simulink library "VSIGenLib"  (R2019b)
settings: Solver=VariableStepAuto  StartTime=0.0  StopTime=10.0  RelTol=1e-3
PostLoadFcn:
  | , if any(exist('dsrtsu_mdlpostloadfcn', 'file') ~= 0), dsrtsu_mdlpostloadfcn('Execute', bdroot); end,
undefined symbols (not defined in the file or in its folder): LIDAR, Ts_hil
libraries: simulink x76, $bdroot x46, etargetslib x30, ASCGenLib x26, dsmpblib x6
(part 3 of 3)

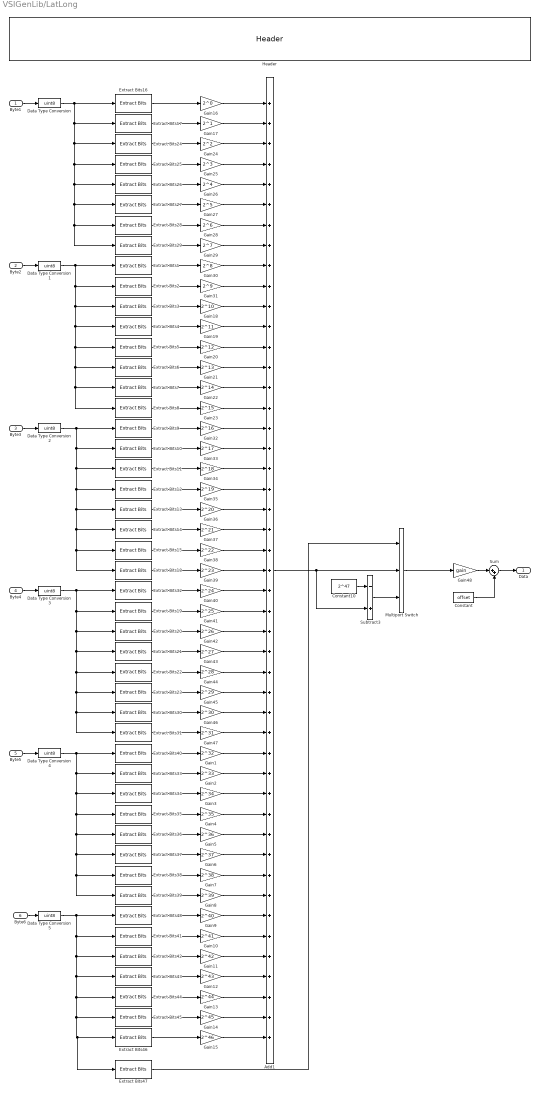
== system VSIGenLib/LatLong ==
  Byte1 : Inport
  Byte2 : Inport  Port=2
  Byte3 : Inport  Port=3
  Byte4 : Inport  Port=4
  Byte5 : Inport  Port=5
  Byte6 : Inport  Port=6
  Add1 : Sum  Inputs=+++++++++++++++++++++++++++++++++++++++++++++++
  Constant : Constant  Value=offset  OutDataTypeStr=double
  Constant10 : Constant  Value=2^47
  Data Type Conversion{,1..5} (6 alike) : DataTypeConversion  OutDataTypeStr=uint8
  Extract Bits{1,9,16,32,40,48} (6 alike) : simulink/Logic and Bit Operations/Extract Bits  bitsToExtract=Range of bits  numBits=8  bitIdxRange=0  outScalingMode=Treat bit field as an integer
      settings: SourceProductName=Simulink
  Extract Bits{2,10,17,19,33,41} (6 alike) : simulink/Logic and Bit Operations/Extract Bits  bitsToExtract=Range of bits  numBits=8  bitIdxRange=1  outScalingMode=Treat bit field as an integer
      settings: SourceProductName=Simulink
  Extract Bits{3,11,20,24,34,42} (6 alike) : simulink/Logic and Bit Operations/Extract Bits  bitsToExtract=Range of bits  numBits=8  bitIdxRange=2  outScalingMode=Treat bit field as an integer
      settings: SourceProductName=Simulink
  Extract Bits{4,12,21,25,35,43} (6 alike) : simulink/Logic and Bit Operations/Extract Bits  bitsToExtract=Range of bits  numBits=8  bitIdxRange=3  outScalingMode=Treat bit field as an integer
      settings: SourceProductName=Simulink
  Extract Bits{5,13,22,26,36,44} (6 alike) : simulink/Logic and Bit Operations/Extract Bits  bitsToExtract=Range of bits  numBits=8  bitIdxRange=4  outScalingMode=Treat bit field as an integer
      settings: SourceProductName=Simulink
  Extract Bits{6,14,23,27,37,45} (6 alike) : simulink/Logic and Bit Operations/Extract Bits  bitsToExtract=Range of bits  numBits=8  bitIdxRange=5  outScalingMode=Treat bit field as an integer
      settings: SourceProductName=Simulink
  Extract Bits{7,15,28,30,38,46} (6 alike) : simulink/Logic and Bit Operations/Extract Bits  bitsToExtract=Range of bits  numBits=8  bitIdxRange=6  outScalingMode=Treat bit field as an integer
      settings: SourceProductName=Simulink
  Extract Bits{8,18,29,31,39,47} (6 alike) : simulink/Logic and Bit Operations/Extract Bits  bitsToExtract=Range of bits  numBits=8  bitIdxRange=7  outScalingMode=Treat bit field as an integer
      settings: SourceProductName=Simulink
  Gain1 : Gain  Gain=2^32  ParamDataTypeStr=double  OutDataTypeStr=double
  Gain10 : Gain  Gain=2^41  ParamDataTypeStr=double  OutDataTypeStr=double
  Gain11 : Gain  Gain=2^42  ParamDataTypeStr=double  OutDataTypeStr=double
  Gain12 : Gain  Gain=2^43  ParamDataTypeStr=double  OutDataTypeStr=double
  Gain13 : Gain  Gain=2^44  ParamDataTypeStr=double  OutDataTypeStr=double
  Gain14 : Gain  Gain=2^45  ParamDataTypeStr=double  OutDataTypeStr=double
  Gain15 : Gain  Gain=2^46  ParamDataTypeStr=double  OutDataTypeStr=double
  Gain16 : Gain  Gain=2^0  ParamDataTypeStr=double  OutDataTypeStr=double
  Gain17 : Gain  Gain=2^1  ParamDataTypeStr=double  OutDataTypeStr=double
  Gain18 : Gain  Gain=2^10  ParamDataTypeStr=double  OutDataTypeStr=double
  Gain19 : Gain  Gain=2^11  ParamDataTypeStr=double  OutDataTypeStr=double
  Gain2 : Gain  Gain=2^33  ParamDataTypeStr=double  OutDataTypeStr=double
  Gain20 : Gain  Gain=2^12  ParamDataTypeStr=double  OutDataTypeStr=double
  Gain21 : Gain  Gain=2^13  ParamDataTypeStr=double  OutDataTypeStr=double
  Gain22 : Gain  Gain=2^14  ParamDataTypeStr=double  OutDataTypeStr=double
  Gain23 : Gain  Gain=2^15  ParamDataTypeStr=double  OutDataTypeStr=double
  Gain24 : Gain  Gain=2^2  ParamDataTypeStr=double  OutDataTypeStr=double
  Gain25 : Gain  Gain=2^3  ParamDataTypeStr=double  OutDataTypeStr=double
  Gain26 : Gain  Gain=2^4  ParamDataTypeStr=double  OutDataTypeStr=double
  Gain27 : Gain  Gain=2^5  ParamDataTypeStr=double  OutDataTypeStr=double
  Gain28 : Gain  Gain=2^6  ParamDataTypeStr=double  OutDataTypeStr=double
  Gain29 : Gain  Gain=2^7  ParamDataTypeStr=double  OutDataTypeStr=double
  Gain3 : Gain  Gain=2^34  ParamDataTypeStr=double  OutDataTypeStr=double
  Gain30 : Gain  Gain=2^8  ParamDataTypeStr=double  OutDataTypeStr=double
  Gain31 : Gain  Gain=2^9  ParamDataTypeStr=double  OutDataTypeStr=double
  Gain32 : Gain  Gain=2^16  ParamDataTypeStr=double  OutDataTypeStr=double
  Gain33 : Gain  Gain=2^17  ParamDataTypeStr=double  OutDataTypeStr=double
  Gain34 : Gain  Gain=2^18  ParamDataTypeStr=double  OutDataTypeStr=double
  Gain35 : Gain  Gain=2^19  ParamDataTypeStr=double  OutDataTypeStr=double
  Gain36 : Gain  Gain=2^20  ParamDataTypeStr=double  OutDataTypeStr=double
  Gain37 : Gain  Gain=2^21  ParamDataTypeStr=double  OutDataTypeStr=double
  Gain38 : Gain  Gain=2^22  ParamDataTypeStr=double  OutDataTypeStr=double
  Gain39 : Gain  Gain=2^23  ParamDataTypeStr=double  OutDataTypeStr=double
  Gain4 : Gain  Gain=2^35  ParamDataTypeStr=double  OutDataTypeStr=double
  Gain40 : Gain  Gain=2^24  ParamDataTypeStr=double  OutDataTypeStr=double
  Gain41 : Gain  Gain=2^25  ParamDataTypeStr=double  OutDataTypeStr=double
  Gain42 : Gain  Gain=2^26  ParamDataTypeStr=double  OutDataTypeStr=double
  Gain43 : Gain  Gain=2^27  ParamDataTypeStr=double  OutDataTypeStr=double
  Gain44 : Gain  Gain=2^28  ParamDataTypeStr=double  OutDataTypeStr=double
  Gain45 : Gain  Gain=2^29  ParamDataTypeStr=double  OutDataTypeStr=double
  Gain46 : Gain  Gain=2^30  ParamDataTypeStr=double  OutDataTypeStr=double
  Gain47 : Gain  Gain=2^31  ParamDataTypeStr=double  OutDataTypeStr=double
  Gain48 : Gain  Gain=gain  ParamDataTypeStr=double  OutDataTypeStr=double
  Gain5 : Gain  Gain=2^36  ParamDataTypeStr=double  OutDataTypeStr=double
  Gain6 : Gain  Gain=2^37  ParamDataTypeStr=double  OutDataTypeStr=double
  Gain7 : Gain  Gain=2^38  ParamDataTypeStr=double  OutDataTypeStr=double
  Gain8 : Gain  Gain=2^39  ParamDataTypeStr=double  OutDataTypeStr=double
  Gain9 : Gain  Gain=2^40  ParamDataTypeStr=double  OutDataTypeStr=double
  Header : $bdroot/Header  not=''
  Multiport Switch : MultiPortSwitch  DataPortOrder=Zero-based contiguous  Inputs=2  zeroidx=on
  Subtract3 : Sum  Inputs=-+
  Sum : Sum  Inputs=|++
  Data : Outport  VectorParamsAs1DForOutWhenUnconnected=off
  wires:
  Extract Bits16/1 -> Gain16/1
  Extract Bits26/1 -> Gain26/1
  Extract Bits27/1 -> Gain27/1
  Extract Bits28/1 -> Gain28/1
  Extract Bits29/1 -> Gain29/1
  Extract Bits1/1 -> Gain30/1
  Extract Bits2/1 -> Gain31/1
  Extract Bits3/1 -> Gain18/1
  Extract Bits4/1 -> Gain19/1
  Extract Bits5/1 -> Gain20/1
  Extract Bits6/1 -> Gain21/1
  Extract Bits7/1 -> Gain22/1
  Extract Bits8/1 -> Gain23/1
  Gain16/1 -> Add1/1
  Gain17/1 -> Add1/2
  Gain24/1 -> Add1/3
  Gain25/1 -> Add1/4
  Gain26/1 -> Add1/5
  Gain27/1 -> Add1/6
  Gain28/1 -> Add1/7
  Gain29/1 -> Add1/8
  Gain30/1 -> Add1/9
  Gain31/1 -> Add1/10
  Gain18/1 -> Add1/11
  Gain19/1 -> Add1/12
  Gain20/1 -> Add1/13
  Gain21/1 -> Add1/14
  Gain22/1 -> Add1/15
  Gain23/1 -> Add1/16
  Extract Bits19/1 -> Gain41/1
  Extract Bits10/1 -> Gain33/1
  Extract Bits20/1 -> Gain42/1
  Extract Bits9/1 -> Gain32/1
  Extract Bits21/1 -> Gain43/1
  Extract Bits11/1 -> Gain34/1
  Extract Bits22/1 -> Gain44/1
  Extract Bits23/1 -> Gain45/1
  Extract Bits30/1 -> Gain46/1
  Extract Bits12/1 -> Gain35/1
  Extract Bits13/1 -> Gain36/1
  Extract Bits14/1 -> Gain37/1
  Extract Bits15/1 -> Gain38/1
  Extract Bits18/1 -> Gain39/1
  Extract Bits32/1 -> Gain40/1
  Extract Bits31/1 -> Gain47/1
  Gain32/1 -> Add1/17
  Gain33/1 -> Add1/18
  Gain34/1 -> Add1/19
  Gain35/1 -> Add1/20
  Gain36/1 -> Add1/21
  Gain37/1 -> Add1/22
  Gain38/1 -> Add1/23
  Gain39/1 -> Add1/24
  Gain40/1 -> Add1/25
  Gain41/1 -> Add1/26
  Gain42/1 -> Add1/27
  Gain43/1 -> Add1/28
  Gain44/1 -> Add1/29
  Gain45/1 -> Add1/30
  Gain46/1 -> Add1/31
  Gain47/1 -> Add1/32
  Byte1/1 -> Data Type Conversion/1
  Byte2/1 -> Data Type Conversion1/1
  Byte3/1 -> Data Type Conversion2/1
  Data Type Conversion3/1 -> Extract Bits19/1, Extract Bits22/1, Extract Bits23/1, Extract Bits30/1, Extract Bits31/1, Extract Bits21/1, Extract Bits20/1, Extract Bits32/1
  Extract Bits33/1 -> Gain2/1
  Extract Bits34/1 -> Gain3/1
  Extract Bits35/1 -> Gain4/1
  Extract Bits36/1 -> Gain5/1
  Extract Bits37/1 -> Gain6/1
  Extract Bits38/1 -> Gain7/1
  Extract Bits40/1 -> Gain1/1
  Extract Bits39/1 -> Gain8/1
  Gain1/1 -> Add1/33
  Gain2/1 -> Add1/34
  Gain3/1 -> Add1/35
  Gain4/1 -> Add1/36
  Gain5/1 -> Add1/37
  Gain6/1 -> Add1/38
  Gain7/1 -> Add1/39
  Gain8/1 -> Add1/40
  Data Type Conversion4/1 -> Extract Bits34/1, Extract Bits35/1, Extract Bits39/1, Extract Bits38/1, Extract Bits37/1, Extract Bits36/1, Extract Bits33/1, Extract Bits40/1
  Extract Bits41/1 -> Gain10/1
  Extract Bits42/1 -> Gain11/1
  Extract Bits43/1 -> Gain12/1
  Extract Bits44/1 -> Gain13/1
  Extract Bits45/1 -> Gain14/1
  Extract Bits46/1 -> Gain15/1
  Extract Bits48/1 -> Gain9/1
  Data Type Conversion5/1 -> Extract Bits48/1, Extract Bits41/1, Extract Bits44/1, Extract Bits45/1, Extract Bits47/1, Extract Bits46/1, Extract Bits43/1, Extract Bits42/1
  Gain15/1 -> Add1/47
  Gain14/1 -> Add1/46
  Gain13/1 -> Add1/45
  Gain12/1 -> Add1/44
  Gain10/1 -> Add1/42
  Gain11/1 -> Add1/43
  Gain9/1 -> Add1/41
  Constant10/1 -> Subtract3/1
  Add1/1 -> Subtract3/2, Multiport Switch/2
  Extract Bits17/1 -> Gain17/1
  Extract Bits25/1 -> Gain25/1
  Extract Bits24/1 -> Gain24/1
  Gain48/1 -> Sum/1
  Constant/1 -> Sum/2
  Multiport Switch/1 -> Gain48/1
  Sum/1 -> Data/1
  Extract Bits47/1 -> Multiport Switch/1
  Subtract3/1 -> Multiport Switch/3
  Data Type Conversion/1 -> Extract Bits17/1, Extract Bits24/1, Extract Bits25/1, Extract Bits27/1, Extract Bits28/1, Extract Bits29/1, Extract Bits26/1, Extract Bits16/1
  Data Type Conversion1/1 -> Extract Bits2/1, Extract Bits3/1, Extract Bits4/1, Extract Bits5/1, Extract Bits6/1, Extract Bits7/1, Extract Bits8/1, Extract Bits1/1
  Data Type Conversion2/1 -> Extract Bits10/1, Extract Bits11/1, Extract Bits12/1, Extract Bits13/1, Extract Bits14/1, Extract Bits15/1, Extract Bits18/1, Extract Bits9/1
  Byte4/1 -> Data Type Conversion3/1
  Byte5/1 -> Data Type Conversion4/1
  Byte6/1 -> Data Type Conversion5/1

== system VSIGenLib/ManualOverride ==
  Data : Inport
  Header : $bdroot/Header  not=''
  Multiport Switch : MultiPortSwitch  Inputs=2
  OvrEnbl : Constant  OutDataTypeStr=boolean
  OvrVal : Constant  Value=0
  "Data " : Outport  VectorParamsAs1DForOutWhenUnconnected=off
  wires:
  Multiport Switch/1 -> "Data "/1
  Data/1 -> Multiport Switch/2
  OvrEnbl/1 -> Multiport Switch/1
  OvrVal/1 -> Multiport Switch/3

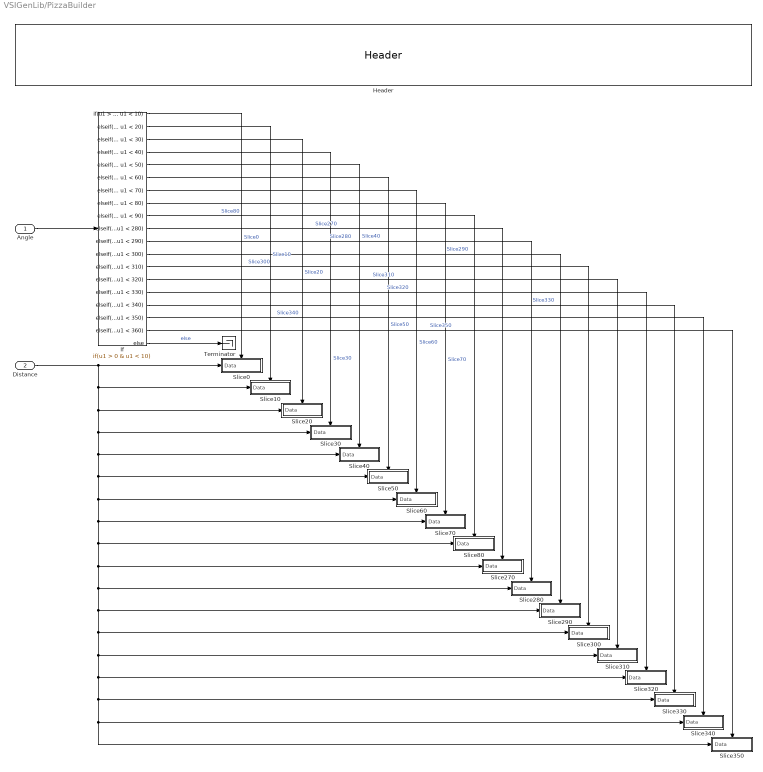
== system VSIGenLib/PizzaBuilder ==
  Angle : Inport
  Distance : Inport  Port=2
  Header : $bdroot/Header  not=''
  If : If  IfExpression=u1 > 0 & u1 < 10  ElseIfExpressions="u1 > 10 & u1 < 20, u1 > 20 & u1 < 30, u1 > 30 & u1 < 40, u1 > 40 & u1 < 50, u1 > 50 & u1 < 60, u1 > 60 & u1 < 70, u1 > 70 & u1 < 80, u1 > 80 & u1 < 90, u1 > 270 & u1 < 280,  u1 > 280 & u1 < 290,  u1 > 290 & u1 < 300,  u1 > 300 & u1 < 310,  u1 > 310 & u1 < 320, u1 > 320 & u1 < 330, u1 > 330 & u1 < 340, u1 > 340 & u1 < 350,  u1 > 350 & u1 < 360"
  Slice0 : Subsystem
  Slice10 : Subsystem
  Slice20 : Subsystem
  Slice270 : Subsystem
  Slice280 : Subsystem
  Slice290 : Subsystem
  Slice30 : Subsystem
  Slice300 : Subsystem
  Slice310 : Subsystem
  Slice320 : Subsystem
  Slice330 : Subsystem
  Slice340 : Subsystem
  Slice350 : Subsystem
  Slice40 : Subsystem
  Slice50 : Subsystem
  Slice60 : Subsystem
  Slice70 : Subsystem
  Slice80 : Subsystem
  Terminator : Terminator
  wires:
  If/19 -> Terminator/1  "else"
  If/18 -> Slice350/Action  "Slice350"
  If/17 -> Slice340/Action  "Slice340"
  If/16 -> Slice330/Action  "Slice330"
  If/15 -> Slice320/Action  "Slice320"
  If/14 -> Slice310/Action  "Slice310"
  If/13 -> Slice300/Action  "Slice300"
  If/12 -> Slice290/Action  "Slice290"
  If/11 -> Slice280/Action  "Slice280"
  If/10 -> Slice270/Action  "Slice270"
  If/9 -> Slice80/Action  "Slice80"
  If/8 -> Slice70/Action  "Slice70"
  If/7 -> Slice60/Action  "Slice60"
  If/6 -> Slice50/Action  "Slice50"
  If/5 -> Slice40/Action  "Slice40"
  If/4 -> Slice30/Action  "Slice30"
  If/3 -> Slice20/Action  "Slice20"
  If/2 -> Slice10/Action  "Slice10"
  If/1 -> Slice0/Action  "Slice0"
  Angle/1 -> If/1
  Distance/1 -> Slice350/1(Data), Slice340/1(Data), Slice330/1(Data), Slice320/1(Data), Slice310/1(Data), Slice300/1(Data), Slice290/1(Data), Slice280/1(Data), Slice270/1(Data), Slice80/1(Data), Slice70/1(Data), Slice60/1(Data), Slice50/1(Data), Slice40/1(Data), Slice30/1(Data), Slice20/1(Data), Slice10/1(Data), Slice0/1(Data)

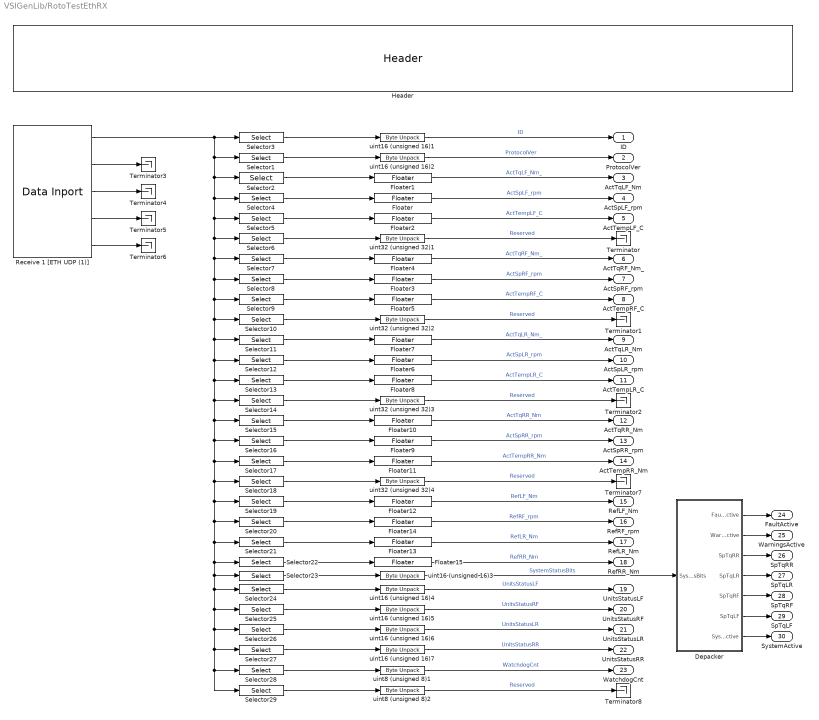
== system VSIGenLib/RotoTestEthRX ==
  Depacker : Subsystem
  Floater{,1..15} (16 alike) : $bdroot/Floater  SystemSampleTime=-1  Latency=0  AutoFrameSizeCalculation=off
  Header : $bdroot/Header  not=''
  Receive 1 [ETH UDP (1)] : dsmpblib/Data Inport  Priority=10000
      settings: SourceProductName=dSPACE Model Interface Blockset
  Selector1 : Selector  IndexMode=Zero-based  InputPortWidth=96  IndexOptions=Index vector (dialog)  Indices=[3 2]  OutputSizes=1
  Selector10 : Selector  IndexMode=Zero-based  InputPortWidth=96  IndexOptions=Index vector (dialog)  Indices=[35 34 33 32]  OutputSizes=1
  Selector11 : Selector  IndexMode=Zero-based  InputPortWidth=96  IndexOptions=Index vector (dialog)  Indices=[39 38 37 36]  OutputSizes=1
  Selector12 : Selector  IndexMode=Zero-based  InputPortWidth=96  IndexOptions=Index vector (dialog)  Indices=[43 42 41 40]  OutputSizes=1
  Selector13 : Selector  IndexMode=Zero-based  InputPortWidth=96  IndexOptions=Index vector (dialog)  Indices=[47 46 45 44]  OutputSizes=1
  Selector14 : Selector  IndexMode=Zero-based  InputPortWidth=96  IndexOptions=Index vector (dialog)  Indices=[51 50 49 48]  OutputSizes=1
  Selector15 : Selector  IndexMode=Zero-based  InputPortWidth=96  IndexOptions=Index vector (dialog)  Indices=[55 54 53 52]  OutputSizes=1
  Selector16 : Selector  IndexMode=Zero-based  InputPortWidth=96  IndexOptions=Index vector (dialog)  Indices=[59 58 57 56]  OutputSizes=1
  Selector17 : Selector  IndexMode=Zero-based  InputPortWidth=96  IndexOptions=Index vector (dialog)  Indices=[63 62 61 60]  OutputSizes=1
  Selector18 : Selector  IndexMode=Zero-based  InputPortWidth=96  IndexOptions=Index vector (dialog)  Indices=[67 66 65 64]  OutputSizes=1
  Selector19 : Selector  IndexMode=Zero-based  InputPortWidth=96  IndexOptions=Index vector (dialog)  Indices=[71 70 69 68]  OutputSizes=1
  Selector2 : Selector  IndexMode=Zero-based  InputPortWidth=96  IndexOptions=Index vector (dialog)  Indices=[7 6 5 4]  OutputSizes=1
  Selector20 : Selector  IndexMode=Zero-based  InputPortWidth=96  IndexOptions=Index vector (dialog)  Indices=[75 74 73 72]  OutputSizes=1
  Selector21 : Selector  IndexMode=Zero-based  InputPortWidth=96  IndexOptions=Index vector (dialog)  Indices=[79 78 77 76]  OutputSizes=1
  Selector22 : Selector  IndexMode=Zero-based  InputPortWidth=96  IndexOptions=Index vector (dialog)  Indices=[83 82 81 80]  OutputSizes=1
  Selector23 : Selector  IndexMode=Zero-based  InputPortWidth=96  IndexOptions=Index vector (dialog)  Indices=[85 84]  OutputSizes=1
  Selector24 : Selector  IndexMode=Zero-based  InputPortWidth=96  IndexOptions=Index vector (dialog)  Indices=[87 86]  OutputSizes=1
  Selector25 : Selector  IndexMode=Zero-based  InputPortWidth=96  IndexOptions=Index vector (dialog)  Indices=[89 88]  OutputSizes=1
  Selector26 : Selector  IndexMode=Zero-based  InputPortWidth=96  IndexOptions=Index vector (dialog)  Indices=[91 90]  OutputSizes=1
  Selector27 : Selector  IndexMode=Zero-based  InputPortWidth=96  IndexOptions=Index vector (dialog)  Indices=[93 92]  OutputSizes=1
  Selector28 : Selector  IndexMode=Zero-based  InputPortWidth=96  IndexOptions=Index vector (dialog)  Indices=[94]  OutputSizes=1
  Selector29 : Selector  IndexMode=Zero-based  InputPortWidth=96  IndexOptions=Index vector (dialog)  Indices=[95]  OutputSizes=1
  Selector3 : Selector  IndexMode=Zero-based  InputPortWidth=96  IndexOptions=Index vector (dialog)  Indices=[1 0]  OutputSizes=1
  Selector4 : Selector  IndexMode=Zero-based  InputPortWidth=96  IndexOptions=Index vector (dialog)  Indices=[11 10 9 8]  OutputSizes=1
  Selector5 : Selector  IndexMode=Zero-based  InputPortWidth=96  IndexOptions=Index vector (dialog)  Indices=[15 14 13 12]  OutputSizes=1
  Selector6 : Selector  IndexMode=Zero-based  InputPortWidth=96  IndexOptions=Index vector (dialog)  Indices=[19 18 17 16]  OutputSizes=1
  Selector7 : Selector  IndexMode=Zero-based  InputPortWidth=96  IndexOptions=Index vector (dialog)  Indices=[23 22 21 20]  OutputSizes=1
  Selector8 : Selector  IndexMode=Zero-based  InputPortWidth=96  IndexOptions=Index vector (dialog)  Indices=[27 26 25 24]  OutputSizes=1
  Selector9 : Selector  IndexMode=Zero-based  InputPortWidth=96  IndexOptions=Index vector (dialog)  Indices=[31 30 29 28]  OutputSizes=1
  Terminator{,1..8} (9 alike) : Terminator
  uint16 (unsigned 16){1..7} (7 alike) : etargetslib/Byte Unpack  dimensions={[1]}  datatypes={'uint16'}  byteAlign=1
      settings: SourceProductName=MATLAB Coder
  uint32 (unsigned 32){1..4} (4 alike) : etargetslib/Byte Unpack  dimensions={[1]}  datatypes={'uint32'}  byteAlign=1
      settings: SourceProductName=MATLAB Coder
  uint8 (unsigned 8)1 : etargetslib/Byte Unpack  dimensions={[1]}  datatypes={'uint8'}  byteAlign=1
      settings: SourceProductName=MATLAB Coder
  uint8 (unsigned 8)2 : etargetslib/Byte Unpack  dimensions={[1]}  datatypes={'uint8'}  byteAlign=1
      settings: SourceProductName=MATLAB Coder
  ID : Outport
  ProtocolVer : Outport  Port=2
  ActTqLF_Nm : Outport  Port=3
  ActSpLF_rpm : Outport  Port=4
  ActTempLF_C : Outport  Port=5
  ActTqRF_Nm_ : Outport  Port=6
  ActSpRF_rpm : Outport  Port=7
  ActTempRF_C : Outport  Port=8
  ActTqLR_Nm : Outport  Port=9
  ActSpLR_rpm : Outport  Port=10
  ActTempLR_C : Outport  Port=11
  ActTqRR_Nm : Outport  Port=12
  ActSpRR_rpm : Outport  Port=13
  ActTempRR_Nm : Outport  Port=14
  RefLF_Nm : Outport  Port=15
  RefRF_rpm : Outport  Port=16
  RefLR_Nm : Outport  Port=17
  RefRR_Nm : Outport  Port=18
  UnitsStatusLF : Outport  Port=19
  UnitsStatusRF : Outport  Port=20
  UnitsStatusLR : Outport  Port=21
  UnitsStatusRR : Outport  Port=22
  WatchdogCnt : Outport  Port=23
  FaultActive : Outport  Port=24
  WarningsActive : Outport  Port=25
  SpTqRR : Outport  Port=26
  SpTqLR : Outport  Port=27
  SpTqRF : Outport  Port=28
  SpTqLF : Outport  Port=29
  SystemActive : Outport  Port=30
  wires:
  Depacker/7(SystemActive) -> SystemActive/1
  Depacker/5(SpTqRF) -> SpTqRF/1
  Depacker/1(FaultActive) -> FaultActive/1
  Depacker/2(WarningsActive) -> WarningsActive/1
  Depacker/3(SpTqRR) -> SpTqRR/1
  Depacker/4(SpTqLR) -> SpTqLR/1
  Depacker/6(SpTqLF) -> SpTqLF/1
  Floater5/1 -> ActTempRF_C/1  "ActTempRF_C"
  uint32 (unsigned 32)2/1 -> Terminator1/1  "Reserved"
  Floater/1 -> ActSpLF_rpm/1  "ActSpLF_rpm"
  uint32 (unsigned 32)1/1 -> Terminator/1  "Reserved"
  uint16 (unsigned 16)1/1 -> ID/1  "ID"
  Floater15/1 -> RefRR_Nm/1  "RefRR_Nm"
  uint8 (unsigned 8)1/1 -> WatchdogCnt/1  "WatchdogCnt"
  Floater14/1 -> RefRF_rpm/1  "RefRF_rpm"
  uint16 (unsigned 16)5/1 -> UnitsStatusRF/1  "UnitsStatusRF"
  uint32 (unsigned 32)3/1 -> Terminator2/1  "Reserved"
  Floater9/1 -> ActSpRR_rpm/1  "ActSpRR_rpm"
  Floater1/1 -> ActTqLF_Nm/1  "ActTqLF_Nm_"
  Floater2/1 -> ActTempLF_C/1  "ActTempLF_C"
  Floater12/1 -> RefLF_Nm/1  "RefLF_Nm"
  Floater7/1 -> ActTqLR_Nm/1  "ActTqLR_Nm_"
  uint16 (unsigned 16)2/1 -> ProtocolVer/1  "ProtocolVer"
  Selector24/1 -> uint16 (unsigned 16)4/1
  Selector7/1 -> Floater4/1
  Selector8/1 -> Floater3/1
  uint16 (unsigned 16)7/1 -> UnitsStatusRR/1  "UnitsStatusRR"
  Selector22/1 -> Floater15/1
  Selector18/1 -> uint32 (unsigned 32)4/1
  Selector12/1 -> Floater6/1
  Selector23/1 -> uint16 (unsigned 16)3/1
  uint16 (unsigned 16)6/1 -> UnitsStatusLR/1  "UnitsStatusLR"
  Selector17/1 -> Floater11/1
  Receive 1 [ETH UDP (1)]/3 -> Terminator4/1
  uint16 (unsigned 16)4/1 -> UnitsStatusLF/1  "UnitsStatusLF"
  Selector27/1 -> uint16 (unsigned 16)7/1
  Floater13/1 -> RefLR_Nm/1  "RefLR_Nm"
  Selector14/1 -> uint32 (unsigned 32)3/1
  Selector2/1 -> Floater1/1
  Selector13/1 -> Floater8/1
  Selector26/1 -> uint16 (unsigned 16)6/1
  Selector6/1 -> uint32 (unsigned 32)1/1
  uint16 (unsigned 16)3/1 -> Depacker/1(SysStsBits)  "SystemStatusBits"
  uint32 (unsigned 32)4/1 -> Terminator7/1  "Reserved"
  Floater3/1 -> ActSpRF_rpm/1  "ActSpRF_rpm"
  Receive 1 [ETH UDP (1)]/2 -> Terminator3/1
  Selector25/1 -> uint16 (unsigned 16)5/1
  Floater4/1 -> ActTqRF_Nm_/1  "ActTqRF_Nm_"
  uint8 (unsigned 8)2/1 -> Terminator8/1  "Reserved"
  Floater11/1 -> ActTempRR_Nm/1  "ActTempRR_Nm"
  Floater6/1 -> ActSpLR_rpm/1  "ActSpLR_rpm"
  Selector20/1 -> Floater14/1
  Selector9/1 -> Floater5/1
  Selector5/1 -> Floater2/1
  Selector15/1 -> Floater10/1
  Selector16/1 -> Floater9/1
  Floater8/1 -> ActTempLR_C/1  "ActTempLR_C"
  Selector3/1 -> uint16 (unsigned 16)1/1
  Receive 1 [ETH UDP (1)]/4 -> Terminator5/1
  Selector28/1 -> uint8 (unsigned 8)1/1
  Selector29/1 -> uint8 (unsigned 8)2/1
  Selector21/1 -> Floater13/1
  Receive 1 [ETH UDP (1)]/1 -> Selector7/1, Selector8/1, Selector9/1, Selector10/1, Selector11/1, Selector12/1, Selector13/1, Selector17/1, Selector18/1, Selector19/1, Selector20/1, Selector21/1, Selector22/1, Selector23/1, Selector25/1, Selector26/1, Selector27/1, Selector29/1, Selector28/1, Selector24/1, Selector16/1, Selector15/1, Selector14/1, Selector6/1, Selector5/1, Selector4/1, Selector2/1, Selector1/1, Selector3/1
  Selector19/1 -> Floater12/1
  Selector10/1 -> uint32 (unsigned 32)2/1
  Selector1/1 -> uint16 (unsigned 16)2/1
  Receive 1 [ETH UDP (1)]/5 -> Terminator6/1
  Selector4/1 -> Floater/1
  Floater10/1 -> ActTqRR_Nm/1  "ActTqRR_Nm"
  Selector11/1 -> Floater7/1

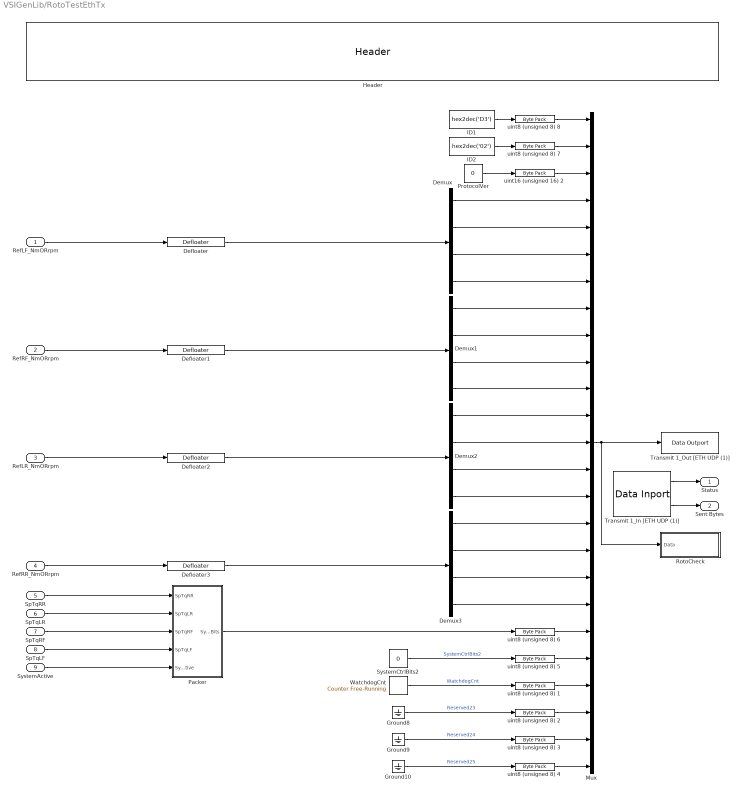
== system VSIGenLib/RotoTestEthTx ==
  RefLF_NmORrpm : Inport
  RefRF_NmORrpm : Inport  Port=2
  RefLR_NmORrpm : Inport  Port=3
  RefRR_NmORrpm : Inport  Port=4
  SpTqRR : Inport  Port=5
  SpTqLR : Inport  Port=6
  SpTqRF : Inport  Port=7
  SpTqLF : Inport  Port=8
  SystemActive : Inport  Port=9
  Defloater{,1..3} (4 alike) : $bdroot/Defloater  SystemSampleTime=-1  Latency=0  AutoFrameSizeCalculation=off
  Demux{,1..3} (4 alike) : Demux
  Ground10 : Ground
  Ground8 : Ground
  Ground9 : Ground
  Header : $bdroot/Header  not=''
  ID1 : Constant  Value=hex2dec('D3')  OutDataTypeStr=uint8
  ID2 : Constant  Value=hex2dec('02')  OutDataTypeStr=uint8
  Mux : Mux  Inputs=25
  Packer : Subsystem
  ProtocolVer : Constant  Value=0  OutDataTypeStr=uint16
  RotoCheck : Subsystem
  SystemCtrlBits2 : Constant  Value=0  OutDataTypeStr=uint8
  Transmit 1_In [ETH UDP (1)] : dsmpblib/Data Inport  Priority=10000
      settings: SourceProductName=dSPACE Model Interface Blockset
  Transmit 1_Out [ETH UDP (1)] : dsmpblib/Data Outport  Priority=-10000
      settings: SourceProductName=dSPACE Model Interface Blockset
  WatchdogCnt : simulink/Sources/Counter Free-Running  NumBits=8  tsamp=-1
  uint16 (unsigned 16) 2 : etargetslib/Byte Pack  datatypes={'uint16'}  byteAlign=1
      settings: SourceProductName=MATLAB Coder
  uint8 (unsigned 8) {1..8} (8 alike) : etargetslib/Byte Pack  datatypes={'uint8'}  byteAlign=1
      settings: SourceProductName=MATLAB Coder
  Status : Outport
  Sent Bytes : Outport  Port=2
  wires:
  Transmit 1_In [ETH UDP (1)]/2 -> Sent Bytes/1
  Transmit 1_In [ETH UDP (1)]/1 -> Status/1
  Packer/1(SystemCtrlBits) -> uint8 (unsigned 8) 6/1
  SystemActive/1 -> Packer/5(SystemActive)
  SpTqLF/1 -> Packer/4(SpTqLF)
  SpTqRF/1 -> Packer/3(SpTqRF)
  SpTqLR/1 -> Packer/2(SpTqLR)
  SpTqRR/1 -> Packer/1(SpTqRR)
  RefLR_NmORrpm/1 -> Defloater2/1
  RefLF_NmORrpm/1 -> Defloater/1
  Demux3/2 -> Mux/17
  Ground8/1 -> uint8 (unsigned 8) 2/1  "Reserved23"
  Demux/2 -> Mux/5
  RefRR_NmORrpm/1 -> Defloater3/1
  uint8 (unsigned 8) 7/1 -> Mux/2
  SystemCtrlBits2/1 -> uint8 (unsigned 8) 5/1  "SystemCtrlBits2"
  Demux3/4 -> Mux/19
  Demux2/4 -> Mux/15
  uint8 (unsigned 8) 8/1 -> Mux/1
  Mux/1 -> Transmit 1_Out [ETH UDP (1)]/1, RotoCheck/1(Data)
  Demux/3 -> Mux/6
  Demux1/2 -> Mux/9
  uint8 (unsigned 8) 6/1 -> Mux/20
  Demux2/3 -> Mux/14
  Demux/4 -> Mux/7
  Demux2/1 -> Mux/12
  Defloater/1 -> Demux/1
  Defloater1/1 -> Demux1/1
  uint16 (unsigned 16) 2/1 -> Mux/3
  uint8 (unsigned 8) 1/1 -> Mux/22
  Demux2/2 -> Mux/13
  uint8 (unsigned 8) 3/1 -> Mux/24
  ProtocolVer/1 -> uint16 (unsigned 16) 2/1
  Demux1/1 -> Mux/8
  Demux3/1 -> Mux/16
  Demux/1 -> Mux/4
  uint8 (unsigned 8) 4/1 -> Mux/25
  ID1/1 -> uint8 (unsigned 8) 8/1
  Ground9/1 -> uint8 (unsigned 8) 3/1  "Reserved24"
  uint8 (unsigned 8) 2/1 -> Mux/23
  Demux1/3 -> Mux/10
  uint8 (unsigned 8) 5/1 -> Mux/21
  Demux3/3 -> Mux/18
  Defloater3/1 -> Demux3/1
  WatchdogCnt/1 -> uint8 (unsigned 8) 1/1  "WatchdogCnt"
  Ground10/1 -> uint8 (unsigned 8) 4/1  "Reserved25"
  Demux1/4 -> Mux/11
  RefRF_NmORrpm/1 -> Defloater1/1
  ID2/1 -> uint8 (unsigned 8) 7/1
  Defloater2/1 -> Demux2/1

== system VSIGenLib/SmartFilter ==
  Slice : Inport
  Tau : Inport  Port=2
  AgeCheck : Stateflow chart  TreatAsAtomicUnit=on
  AgeCheck1 : Stateflow chart  TreatAsAtomicUnit=on
  AgeCheck10 : Stateflow chart  TreatAsAtomicUnit=on
  AgeCheck11 : Stateflow chart  TreatAsAtomicUnit=on
  AgeCheck2 : Stateflow chart  TreatAsAtomicUnit=on
  AgeCheck3 : Stateflow chart  TreatAsAtomicUnit=on
  AgeCheck4 : Stateflow chart  TreatAsAtomicUnit=on
  AgeCheck5 : Stateflow chart  TreatAsAtomicUnit=on
  AgeCheck6 : Stateflow chart  TreatAsAtomicUnit=on
  AgeCheck7 : Stateflow chart  TreatAsAtomicUnit=on
  AgeCheck8 : Stateflow chart  TreatAsAtomicUnit=on
  AgeCheck9 : Stateflow chart  TreatAsAtomicUnit=on
  Demux : Demux  Outputs=12
  FirstOrderFilterTau : $bdroot/FirstOrderFilterTau  SystemSampleTime=-1  Latency=0  AutoFrameSizeCalculation=off
  Header : $bdroot/Header  not=''
  MinMax : MinMax  Inputs=12
  SliceMin : Outport  VectorParamsAs1DForOutWhenUnconnected=off
  wires:
  Demux/1 -> AgeCheck/1(In)
  AgeCheck/1(Out) -> MinMax/1
  Slice/1 -> Demux/1
  MinMax/1 -> FirstOrderFilterTau/1
  Demux/2 -> AgeCheck1/1(In)
  Demux/3 -> AgeCheck2/1(In)
  Demux/4 -> AgeCheck3/1(In)
  Demux/5 -> AgeCheck4/1(In)
  Demux/6 -> AgeCheck5/1(In)
  Demux/7 -> AgeCheck6/1(In)
  Demux/8 -> AgeCheck7/1(In)
  Demux/9 -> AgeCheck8/1(In)
  Demux/10 -> AgeCheck9/1(In)
  Demux/11 -> AgeCheck10/1(In)
  Demux/12 -> AgeCheck11/1(In)
  AgeCheck1/1(Out) -> MinMax/2
  AgeCheck2/1(Out) -> MinMax/3
  AgeCheck3/1(Out) -> MinMax/4
  AgeCheck4/1(Out) -> MinMax/5
  AgeCheck5/1(Out) -> MinMax/6
  AgeCheck6/1(Out) -> MinMax/7
  AgeCheck7/1(Out) -> MinMax/8
  AgeCheck8/1(Out) -> MinMax/9
  AgeCheck9/1(Out) -> MinMax/10
  AgeCheck10/1(Out) -> MinMax/11
  AgeCheck11/1(Out) -> MinMax/12
  Tau/1 -> FirstOrderFilterTau/2
  FirstOrderFilterTau/1 -> SliceMin/1

== system VSIGenLib/Timer ==
  Start : Inport
  Header : $bdroot/Header  not=''
  Memory : Memory  InheritSampleTime=on
  Sum : Sum  Inputs=|++
  Switch : Switch  Criteria=u2 ~= 0
  Ts_hil : Constant  Value=Ts_hil
  Zero : Constant  Value=0
  Timer : Outport  VectorParamsAs1DForOutWhenUnconnected=off
  wires:
  Ts_hil/1 -> Sum/1
  Sum/1 -> Switch/1
  Memory/1 -> Timer/1, Sum/2
  Zero/1 -> Switch/3
  Start/1 -> Switch/2
  Switch/1 -> Memory/1

== system VSIGenLib/PizzaBuilder/Slice0 ==
  Data : Inport
  Action Port : ActionPort  ActionPortLabel=if { }
  CANRxEnblWrite : DataStoreWrite  DataStoreName=Slice0
  Header : ASCGenLib/Header  not=''
  wires:
  Data/1 -> CANRxEnblWrite/1

== system VSIGenLib/PizzaBuilder/Slice10 ==
  Data : Inport
  Action Port : ActionPort  ActionPortLabel=elseif { }
  CANRxEnblWrite : DataStoreWrite  DataStoreName=Slice10
  Header : ASCGenLib/Header  not=''
  wires:
  Data/1 -> CANRxEnblWrite/1

== system VSIGenLib/PizzaBuilder/Slice20 ==
  Data : Inport
  Action Port : ActionPort  ActionPortLabel=elseif { }
  CANRxEnblWrite : DataStoreWrite  DataStoreName=Slice20
  Header : ASCGenLib/Header  not=''
  wires:
  Data/1 -> CANRxEnblWrite/1

== system VSIGenLib/PizzaBuilder/Slice270 ==
  Data : Inport
  Action Port : ActionPort  ActionPortLabel=elseif { }
  CANRxEnblWrite : DataStoreWrite  DataStoreName=Slice270
  Header : ASCGenLib/Header  not=''
  wires:
  Data/1 -> CANRxEnblWrite/1

== system VSIGenLib/PizzaBuilder/Slice280 ==
  Data : Inport
  Action Port : ActionPort  ActionPortLabel=elseif { }
  CANRxEnblWrite : DataStoreWrite  DataStoreName=Slice280
  Header : ASCGenLib/Header  not=''
  wires:
  Data/1 -> CANRxEnblWrite/1

== system VSIGenLib/PizzaBuilder/Slice290 ==
  Data : Inport
  Action Port : ActionPort  ActionPortLabel=elseif { }
  CANRxEnblWrite : DataStoreWrite  DataStoreName=Slice290
  Header : ASCGenLib/Header  not=''
  wires:
  Data/1 -> CANRxEnblWrite/1

== system VSIGenLib/PizzaBuilder/Slice30 ==
  Data : Inport
  Action Port : ActionPort  ActionPortLabel=elseif { }
  CANRxEnblWrite : DataStoreWrite  DataStoreName=Slice30
  Header : ASCGenLib/Header  not=''
  wires:
  Data/1 -> CANRxEnblWrite/1

== system VSIGenLib/PizzaBuilder/Slice300 ==
  Data : Inport
  Action Port : ActionPort  ActionPortLabel=elseif { }
  CANRxEnblWrite : DataStoreWrite  DataStoreName=Slice300
  Header : ASCGenLib/Header  not=''
  wires:
  Data/1 -> CANRxEnblWrite/1

== system VSIGenLib/PizzaBuilder/Slice310 ==
  Data : Inport
  Action Port : ActionPort  ActionPortLabel=elseif { }
  CANRxEnblWrite : DataStoreWrite  DataStoreName=Slice310
  Header : ASCGenLib/Header  not=''
  wires:
  Data/1 -> CANRxEnblWrite/1

== system VSIGenLib/PizzaBuilder/Slice320 ==
  Data : Inport
  Action Port : ActionPort  ActionPortLabel=elseif { }
  CANRxEnblWrite : DataStoreWrite  DataStoreName=Slice320
  Header : ASCGenLib/Header  not=''
  wires:
  Data/1 -> CANRxEnblWrite/1

== system VSIGenLib/PizzaBuilder/Slice330 ==
  Data : Inport
  Action Port : ActionPort  ActionPortLabel=elseif { }
  CANRxEnblWrite : DataStoreWrite  DataStoreName=Slice330
  Header : ASCGenLib/Header  not=''
  wires:
  Data/1 -> CANRxEnblWrite/1

== system VSIGenLib/PizzaBuilder/Slice340 ==
  Data : Inport
  Action Port : ActionPort  ActionPortLabel=elseif { }
  CANRxEnblWrite : DataStoreWrite  DataStoreName=Slice340
  Header : ASCGenLib/Header  not=''
  wires:
  Data/1 -> CANRxEnblWrite/1

== system VSIGenLib/PizzaBuilder/Slice350 ==
  Data : Inport
  Action Port : ActionPort  ActionPortLabel=elseif { }
  CANRxEnblWrite : DataStoreWrite  DataStoreName=Slice350
  Header : ASCGenLib/Header  not=''
  wires:
  Data/1 -> CANRxEnblWrite/1

== system VSIGenLib/PizzaBuilder/Slice40 ==
  Data : Inport
  Action Port : ActionPort  ActionPortLabel=elseif { }
  CANRxEnblWrite : DataStoreWrite  DataStoreName=Slice40
  Header : ASCGenLib/Header  not=''
  wires:
  Data/1 -> CANRxEnblWrite/1

== system VSIGenLib/PizzaBuilder/Slice50 ==
  Data : Inport
  Action Port : ActionPort  ActionPortLabel=elseif { }
  CANRxEnblWrite : DataStoreWrite  DataStoreName=Slice50
  Header : ASCGenLib/Header  not=''
  wires:
  Data/1 -> CANRxEnblWrite/1

== system VSIGenLib/PizzaBuilder/Slice60 ==
  Data : Inport
  Action Port : ActionPort  ActionPortLabel=elseif { }
  CANRxEnblWrite : DataStoreWrite  DataStoreName=Slice60
  Header : ASCGenLib/Header  not=''
  wires:
  Data/1 -> CANRxEnblWrite/1

== system VSIGenLib/PizzaBuilder/Slice70 ==
  Data : Inport
  Action Port : ActionPort  ActionPortLabel=elseif { }
  CANRxEnblWrite : DataStoreWrite  DataStoreName=Slice70
  Header : ASCGenLib/Header  not=''
  wires:
  Data/1 -> CANRxEnblWrite/1

== system VSIGenLib/PizzaBuilder/Slice80 ==
  Data : Inport
  Action Port : ActionPort  ActionPortLabel=elseif { }
  CANRxEnblWrite : DataStoreWrite  DataStoreName=Slice80
  Header : ASCGenLib/Header  not=''
  wires:
  Data/1 -> CANRxEnblWrite/1

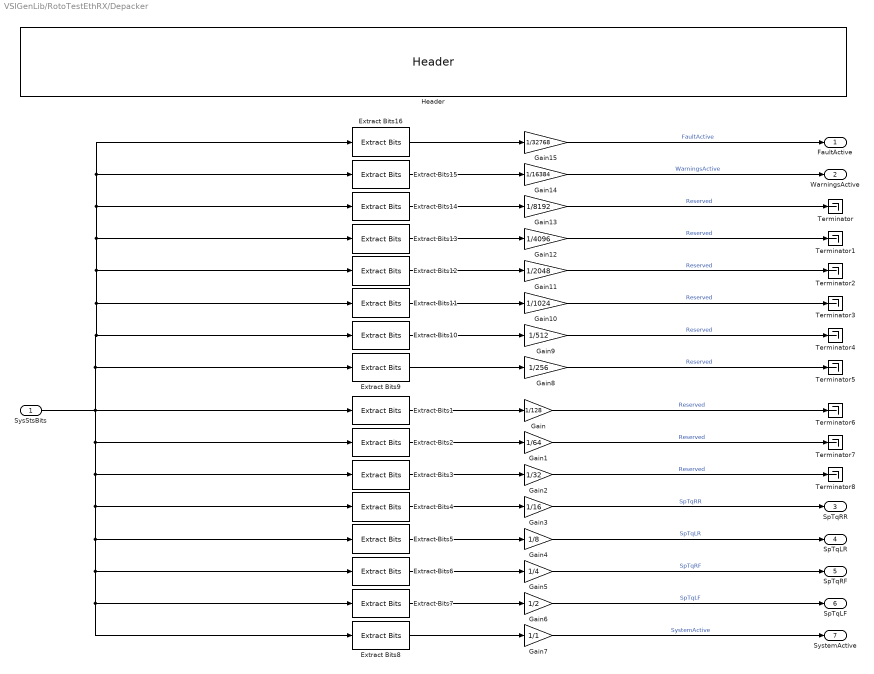
== system VSIGenLib/RotoTestEthRX/Depacker ==
  SysStsBits : Inport
  Extract Bits1 : simulink/Logic and Bit Operations/Extract Bits  bitsToExtract=Range of bits  numBits=8  bitIdxRange=[7]  outScalingMode=Preserve fixed-point scaling
      settings: SourceProductName=Simulink
  Extract Bits10 : simulink/Logic and Bit Operations/Extract Bits  bitsToExtract=Range of bits  numBits=8  bitIdxRange=[9]  outScalingMode=Preserve fixed-point scaling
      settings: SourceProductName=Simulink
  Extract Bits11 : simulink/Logic and Bit Operations/Extract Bits  bitsToExtract=Range of bits  numBits=8  bitIdxRange=[10]  outScalingMode=Preserve fixed-point scaling
      settings: SourceProductName=Simulink
  Extract Bits12 : simulink/Logic and Bit Operations/Extract Bits  bitsToExtract=Range of bits  numBits=8  bitIdxRange=[11]  outScalingMode=Preserve fixed-point scaling
      settings: SourceProductName=Simulink
  Extract Bits13 : simulink/Logic and Bit Operations/Extract Bits  bitsToExtract=Range of bits  numBits=8  bitIdxRange=[12]  outScalingMode=Preserve fixed-point scaling
      settings: SourceProductName=Simulink
  Extract Bits14 : simulink/Logic and Bit Operations/Extract Bits  bitsToExtract=Range of bits  numBits=8  bitIdxRange=[13]  outScalingMode=Preserve fixed-point scaling
      settings: SourceProductName=Simulink
  Extract Bits15 : simulink/Logic and Bit Operations/Extract Bits  bitsToExtract=Range of bits  numBits=8  bitIdxRange=[14]  outScalingMode=Preserve fixed-point scaling
      settings: SourceProductName=Simulink
  Extract Bits16 : simulink/Logic and Bit Operations/Extract Bits  bitsToExtract=Range of bits  numBits=8  bitIdxRange=[15]  outScalingMode=Preserve fixed-point scaling
      settings: SourceProductName=Simulink
  Extract Bits2 : simulink/Logic and Bit Operations/Extract Bits  bitsToExtract=Range of bits  numBits=8  bitIdxRange=[6]  outScalingMode=Preserve fixed-point scaling
      settings: SourceProductName=Simulink
  Extract Bits3 : simulink/Logic and Bit Operations/Extract Bits  bitsToExtract=Range of bits  numBits=8  bitIdxRange=[5]  outScalingMode=Preserve fixed-point scaling
      settings: SourceProductName=Simulink
  Extract Bits4 : simulink/Logic and Bit Operations/Extract Bits  bitsToExtract=Range of bits  numBits=8  bitIdxRange=[4]  outScalingMode=Preserve fixed-point scaling
      settings: SourceProductName=Simulink
  Extract Bits5 : simulink/Logic and Bit Operations/Extract Bits  bitsToExtract=Range of bits  numBits=8  bitIdxRange=[3]  outScalingMode=Preserve fixed-point scaling
      settings: SourceProductName=Simulink
  Extract Bits6 : simulink/Logic and Bit Operations/Extract Bits  bitsToExtract=Range of bits  numBits=8  bitIdxRange=[2]  outScalingMode=Preserve fixed-point scaling
      settings: SourceProductName=Simulink
  Extract Bits7 : simulink/Logic and Bit Operations/Extract Bits  bitsToExtract=Range of bits  numBits=8  bitIdxRange=[1]  outScalingMode=Preserve fixed-point scaling
      settings: SourceProductName=Simulink
  Extract Bits8 : simulink/Logic and Bit Operations/Extract Bits  bitsToExtract=Range of bits  numBits=8  bitIdxRange=[0]  outScalingMode=Preserve fixed-point scaling
      settings: SourceProductName=Simulink
  Extract Bits9 : simulink/Logic and Bit Operations/Extract Bits  bitsToExtract=Range of bits  numBits=8  bitIdxRange=[8]  outScalingMode=Preserve fixed-point scaling
      settings: SourceProductName=Simulink
  Gain : Gain  Gain=1/128
  Gain1 : Gain  Gain=1/64
  Gain10 : Gain  Gain=1/1024
  Gain11 : Gain  Gain=1/2048
  Gain12 : Gain  Gain=1/4096
  Gain13 : Gain  Gain=1/8192
  Gain14 : Gain  Gain=1/16384
  Gain15 : Gain  Gain=1/32768
  Gain2 : Gain  Gain=1/32
  Gain3 : Gain  Gain=1/16
  Gain4 : Gain  Gain=1/8
  Gain5 : Gain  Gain=1/4
  Gain6 : Gain  Gain=1/2
  Gain7 : Gain  Gain=1/1
  Gain8 : Gain  Gain=1/256
  Gain9 : Gain  Gain=1/512
  Header : $bdroot/Header  not=''
  Terminator{,1..8} (9 alike) : Terminator
  FaultActive : Outport
  WarningsActive : Outport  Port=2
  SpTqRR : Outport  Port=3
  SpTqLR : Outport  Port=4
  SpTqRF : Outport  Port=5
  SpTqLF : Outport  Port=6
  SystemActive : Outport  Port=7
  wires:
  Extract Bits10/1 -> Gain9/1
  Extract Bits11/1 -> Gain10/1
  Extract Bits12/1 -> Gain11/1
  Gain10/1 -> Terminator3/1  "Reserved"
  Gain9/1 -> Terminator4/1  "Reserved"
  Gain12/1 -> Terminator1/1  "Reserved"
  Gain11/1 -> Terminator2/1  "Reserved"
  Gain13/1 -> Terminator/1  "Reserved"
  Gain14/1 -> WarningsActive/1  "WarningsActive"
  Gain15/1 -> FaultActive/1  "FaultActive"
  Extract Bits13/1 -> Gain12/1
  Extract Bits14/1 -> Gain13/1
  Extract Bits15/1 -> Gain14/1
  Extract Bits16/1 -> Gain15/1
  Gain8/1 -> Terminator5/1  "Reserved"
  Extract Bits9/1 -> Gain8/1
  Gain7/1 -> SystemActive/1  "SystemActive"
  Gain6/1 -> SpTqLF/1  "SpTqLF"
  Gain5/1 -> SpTqRF/1  "SpTqRF"
  Gain4/1 -> SpTqLR/1  "SpTqLR"
  Gain3/1 -> SpTqRR/1  "SpTqRR"
  Gain1/1 -> Terminator7/1  "Reserved"
  Gain2/1 -> Terminator8/1  "Reserved"
  Gain/1 -> Terminator6/1  "Reserved"
  Extract Bits5/1 -> Gain4/1
  Extract Bits7/1 -> Gain6/1
  SysStsBits/1 -> Extract Bits9/1, Extract Bits10/1, Extract Bits16/1, Extract Bits15/1, Extract Bits14/1, Extract Bits13/1, Extract Bits12/1, Extract Bits11/1, Extract Bits8/1, Extract Bits7/1, Extract Bits6/1, Extract Bits5/1, Extract Bits4/1, Extract Bits3/1, Extract Bits2/1, Extract Bits1/1
  Extract Bits4/1 -> Gain3/1
  Extract Bits1/1 -> Gain/1
  Extract Bits8/1 -> Gain7/1
  Extract Bits3/1 -> Gain2/1
  Extract Bits6/1 -> Gain5/1
  Extract Bits2/1 -> Gain1/1

== system VSIGenLib/RotoTestEthTx/Packer ==
  SpTqRR : Inport
  SpTqLR : Inport  Port=2
  SpTqRF : Inport  Port=3
  SpTqLF : Inport  Port=4
  SystemActive : Inport  Port=5
  Add : Sum  Inputs=++++++++  OutDataTypeStr=uint8
  Bit0 : Gain  OutDataTypeStr=uint8
  Bit1 : Gain  Gain=2  OutDataTypeStr=uint8
  Bit2 : Gain  Gain=4  OutDataTypeStr=Inherit: Inherit via back propagation
  Bit3 : Gain  Gain=8  OutDataTypeStr=uint8
  Bit4 : Gain  Gain=16  OutDataTypeStr=uint8
  Bit5 : Gain  Gain=32  OutDataTypeStr=uint8
  Bit6 : Gain  Gain=64  OutDataTypeStr=uint8
  Bit7 : Gain  Gain=128  OutDataTypeStr=uint8
  Ground11 : Ground
  Header : $bdroot/Header  not=''
  SystemCtrlBits : Outport
  wires:
  SpTqRF/1 -> Bit2/1
  SpTqLF/1 -> Bit1/1
  SpTqRR/1 -> Bit4/1
  SpTqLR/1 -> Bit3/1
  Add/1 -> SystemCtrlBits/1  "SystemCtrlBits"
  Bit0/1 -> Add/8  "SystemActive"
  Bit1/1 -> Add/7  "SpTqLF"
  Bit7/1 -> Add/1  "Reserved"
  SystemActive/1 -> Bit0/1
  Bit4/1 -> Add/4  "SpTqRR"
  Bit6/1 -> Add/2  "Reserved"
  Bit3/1 -> Add/5  "SpTqLR"
  Ground11/1 -> Bit7/1, Bit5/1, Bit6/1  "Reserved"
  Bit5/1 -> Add/3  "Reserved"
  Bit2/1 -> Add/6  "SpTqRF"

== system VSIGenLib/RotoTestEthTx/RotoCheck ==
  Data : Inport
  Header : $bdroot/Header  not=''
  Receive 2 [ETH UDP (1)] : dsmpblib/Data Inport  Priority=10000
      settings: SourceProductName=dSPACE Model Interface Blockset
  Terminator{,1..6} (7 alike) : Terminator
  Transmit 2_In [ETH UDP (1)] : dsmpblib/Data Inport  Priority=10000
      settings: SourceProductName=dSPACE Model Interface Blockset
  Transmit 2_Out [ETH UDP (1)] : dsmpblib/Data Outport  Priority=-10000
      settings: SourceProductName=dSPACE Model Interface Blockset
  wires:
  Transmit 2_In [ETH UDP (1)]/1 -> Terminator/1  "Status"
  Data/1 -> Transmit 2_Out [ETH UDP (1)]/1  "Data"
  Receive 2 [ETH UDP (1)]/3 -> Terminator4/1  "Status"
  Receive 2 [ETH UDP (1)]/5 -> Terminator6/1  "Source Port"
  Receive 2 [ETH UDP (1)]/2 -> Terminator3/1  "Received Bytes"
  Receive 2 [ETH UDP (1)]/1 -> Terminator2/1  "Data"
  Transmit 2_In [ETH UDP (1)]/2 -> Terminator1/1  "Sent Bytes"
  Receive 2 [ETH UDP (1)]/4 -> Terminator5/1  "Source IP Address"

== matlab function VSIGenLib/AngleCalculator ==
  data: azimuth_N input; azimuth_N1 output; azimuth_Next input
function azimuth_N1  = AngleCalc(azimuth_N, azimuth_Next)

if azimuth_Next < azimuth_N
    azimuth_Next = azimuth_Next + 360;
end
azimuth_N1 = azimuth_N + ((azimuth_Next - azimuth_N)/2);
if azimuth_N1 > 360
    azimuth_N1 = azimuth_N1 - 360;
end

end

== stateflow chart VSIGenLib/IHoldValue/HoldVal ==
  state State1
    state Wait
      en:
      Tmr = 0;
      Out = Val;
      du:
      Tmr = Tmr + 1;
    state Pass
      en: Tmr = 0;
      du:
      Out = DIn;
      Tmr = Tmr + 1;
    state Delay
      en:
      Tmr = 0;
      Out = DIn;
      Val = DIn;
      du:
      Tmr = Tmr + 1;
    (default) -> Pass
    Wait -> Pass : [hasChanged(In) &&...
        | In ~= 0 && DIn ~=0]
    Pass -> Delay : [hasChangedTo(In,0)]
    Delay -> Wait : [hasChangedFrom(In,0)]
  state Impact [commented out]
    en:
    Out = 0;
  (default) -> State1
  State1 -> Impact [commented out] : [In == 0 &&...
      | Tmr > 5000]
  Impact -> State1 [commented out] : [In ~=0]
  data: Out output; In input; DIn input; Val local; Tmr local

== stateflow chart VSIGenLib/AgeCheck ==
  state Set
    en:
    Out = In;
    du:
    Cntr = Cntr + 1;
  state Reset
    en:
    Cntr = single(0);
    Out = single(5);
  Set -> Reset [order 2] : [Cntr > 200]
  (default) -> Reset
  Reset -> Set : [hasChanged(In)]
  Set -> Set [order 1] : [hasChanged(In)]
  data: In input single; Out output single; Cntr local single

== stateflow chart VSIGenLib/Toggler2000 ==
  state Off
    en:
    Tmr = 0;
    Switch = false;
    du:
    Tmr = Tmr + 1;
  state On
    en:
    Tmr = 0;
    Switch = true;
    du:
    Tmr = Tmr + 1;
  On -> Off : [hasChangedFrom(Toggle, 0) && ...
      | Tmr > Thr]
  (default) -> Off
  Off -> On : [hasChangedFrom(Toggle, 0) && ...
      | Tmr > Thr]
  data: Toggle input; Switch output; Tmr local; Thr input

== stateflow chart VSIGenLib/Toggler9001 ==
  state Off
    en:
    Switch = false;
  state On
    en:
    Switch = true;
  On -> Off : [hasChangedFrom(Toggle, 0) && ...
      | after(thr, sec)]
  (default) -> Off
  Off -> On : [hasChangedFrom(Toggle, 0) && ...
      | after(thr, sec) ]
  data: Toggle input; thr input; Switch output

== stateflow chart VSIGenLib/SoftstopDM ==
  state InactiveSSDM
    du:
    DMOut = DMIn;
  state SoftStopDM
    en:
    DMOut = 1;
  SoftStopDM -> InactiveSSDM : [after(3, sec)]
  (default) -> InactiveSSDM
  InactiveSSDM -> SoftStopDM : [hasChangedFrom(WPActv, true)]
  data: WPActv input; DMIn input; DMOut output

== stateflow chart VSIGenLib/Toggler9001LE ==
  state Off
    en:
    Switch = false;
  state On
    en:
    Switch = true;
  note: [hasChangedFrom(Toggle, 1)]
  On -> Off [order 1] : [hasChangedFrom(Toggle, 0) && ...
      | after(thr, sec)]
  (default) -> Off
  Off -> (junction 12) : [hasChangedFrom(Toggle, 0) && ...
      | after(thr, sec) ]
  (junction 12) -> On [order 1] : [after(0.5, sec)]
  (junction 12) -> Off [order 2]
  On -> Off [order 2] : [WPBtnDsbl]
  data: Switch output; Toggle input; thr input; WPBtnDsbl input

== stateflow chart VSIGenLib/SmartFilter/AgeCheck ==
  state Set
    en:
    Out = In;
    du:
    Cntr = Cntr + 1;
  state Reset
    en:
    Cntr = single(0);
    Out = single(5);
  Set -> Reset [order 2] : [Cntr > 200]
  (default) -> Reset
  Reset -> Set : [hasChanged(In)]
  Set -> Set [order 1] : [hasChanged(In)]
  data: In input single; Out output single; Cntr local single

== stateflow chart VSIGenLib/SmartFilter/AgeCheck1 ==
  state Set
    en:
    Out = In;
    du:
    Cntr = Cntr + 1;
  state Reset
    en:
    Cntr = single(0);
    Out = single(5);
  Set -> Reset [order 2] : [Cntr > 200]
  (default) -> Reset
  Reset -> Set : [hasChanged(In)]
  Set -> Set [order 1] : [hasChanged(In)]
  data: In input single; Out output single; Cntr local single

== stateflow chart VSIGenLib/SmartFilter/AgeCheck2 ==
  state Set
    en:
    Out = In;
    du:
    Cntr = Cntr + 1;
  state Reset
    en:
    Cntr = single(0);
    Out = single(5);
  Set -> Reset [order 2] : [Cntr > 200]
  (default) -> Reset
  Reset -> Set : [hasChanged(In)]
  Set -> Set [order 1] : [hasChanged(In)]
  data: In input single; Out output single; Cntr local single

== stateflow chart VSIGenLib/SmartFilter/AgeCheck3 ==
  state Set
    en:
    Out = In;
    du:
    Cntr = Cntr + 1;
  state Reset
    en:
    Cntr = single(0);
    Out = single(5);
  Set -> Reset [order 2] : [Cntr > 200]
  (default) -> Reset
  Reset -> Set : [hasChanged(In)]
  Set -> Set [order 1] : [hasChanged(In)]
  data: In input single; Out output single; Cntr local single

== stateflow chart VSIGenLib/SmartFilter/AgeCheck4 ==
  state Set
    en:
    Out = In;
    du:
    Cntr = Cntr + 1;
  state Reset
    en:
    Cntr = single(0);
    Out = single(5);
  Set -> Reset [order 2] : [Cntr > 200]
  (default) -> Reset
  Reset -> Set : [hasChanged(In)]
  Set -> Set [order 1] : [hasChanged(In)]
  data: In input single; Out output single; Cntr local single

== stateflow chart VSIGenLib/SmartFilter/AgeCheck5 ==
  state Set
    en:
    Out = In;
    du:
    Cntr = Cntr + 1;
  state Reset
    en:
    Cntr = single(0);
    Out = single(5);
  Set -> Reset [order 2] : [Cntr > 200]
  (default) -> Reset
  Reset -> Set : [hasChanged(In)]
  Set -> Set [order 1] : [hasChanged(In)]
  data: In input single; Out output single; Cntr local single

== stateflow chart VSIGenLib/SmartFilter/AgeCheck6 ==
  state Set
    en:
    Out = In;
    du:
    Cntr = Cntr + 1;
  state Reset
    en:
    Cntr = single(0);
    Out = single(5);
  Set -> Reset [order 2] : [Cntr > 200]
  (default) -> Reset
  Reset -> Set : [hasChanged(In)]
  Set -> Set [order 1] : [hasChanged(In)]
  data: In input single; Out output single; Cntr local single

== stateflow chart VSIGenLib/SmartFilter/AgeCheck7 ==
  state Set
    en:
    Out = In;
    du:
    Cntr = Cntr + 1;
  state Reset
    en:
    Cntr = single(0);
    Out = single(5);
  Set -> Reset [order 2] : [Cntr > 200]
  (default) -> Reset
  Reset -> Set : [hasChanged(In)]
  Set -> Set [order 1] : [hasChanged(In)]
  data: In input single; Out output single; Cntr local single

== stateflow chart VSIGenLib/SmartFilter/AgeCheck8 ==
  state Set
    en:
    Out = In;
    du:
    Cntr = Cntr + 1;
  state Reset
    en:
    Cntr = single(0);
    Out = single(5);
  Set -> Reset [order 2] : [Cntr > 200]
  (default) -> Reset
  Reset -> Set : [hasChanged(In)]
  Set -> Set [order 1] : [hasChanged(In)]
  data: In input single; Out output single; Cntr local single

== stateflow chart VSIGenLib/SmartFilter/AgeCheck10 ==
  state Set
    en:
    Out = In;
    du:
    Cntr = Cntr + 1;
  state Reset
    en:
    Cntr = single(0);
    Out = single(5);
  Set -> Reset [order 2] : [Cntr > 200]
  (default) -> Reset
  Reset -> Set : [hasChanged(In)]
  Set -> Set [order 1] : [hasChanged(In)]
  data: In input single; Out output single; Cntr local single

== stateflow chart VSIGenLib/SmartFilter/AgeCheck11 ==
  state Set
    en:
    Out = In;
    du:
    Cntr = Cntr + 1;
  state Reset
    en:
    Cntr = single(0);
    Out = single(5);
  Set -> Reset [order 2] : [Cntr > 200]
  (default) -> Reset
  Reset -> Set : [hasChanged(In)]
  Set -> Set [order 1] : [hasChanged(In)]
  data: In input single; Out output single; Cntr local single

== stateflow chart VSIGenLib/SmartFilter/AgeCheck9 ==
  state Set
    en:
    Out = In;
    du:
    Cntr = Cntr + 1;
  state Reset
    en:
    Cntr = single(0);
    Out = single(5);
  Set -> Reset [order 2] : [Cntr > 200]
  (default) -> Reset
  Reset -> Set : [hasChanged(In)]
  Set -> Set [order 1] : [hasChanged(In)]
  data: In input single; Out output single; Cntr local single

== matlab function VSIGenLib/Floater/Floater ==
  data: byte1 input; float32 output; byte2 input; byte3 input; byte4 input
function float32 = floater(byte1, byte2, byte3, byte4)

% This block converts 4 uint8 values into a single floating point number
% based on IEEE-754 standard. By default, byte order is for little endian
% format - use the fliplr function to read big endian.

bytes = zeros(1, 4, 'uint8');
bytes = uint8([byte1, byte2, byte3, byte4]);
bytes = fliplr(bytes);
float32 = zeros(1, 1, 'single');
float32 = typecast(bytes,'single');

== matlab function VSIGenLib/Defloater/Defloater ==
  data: defloatMe input; byte1 output; byte2 output; byte3 output; byte4 output
function [byte1, byte2, byte3, byte4] = defloater(defloatMe)

% This block converts a single floating point number into a 4 byte vector
% based on IEEE-754 standard. By default, byte order is for little endian
% format - use the fliplr function to send big endian.

%float32 = zeros(1, 1, 'single');
float32 = typecast(single(defloatMe), 'uint8');
%float32 = fliplr(float32);
byte1 = float32(1);
byte2 = float32(2);
byte3 = float32(3);
byte4 = float32(4);

== stateflow chart VSIGenLib/Softstop ==
  state InactiveSS
    en:
    SSActv = 0;
  state SoftStop
    en:
    SSActv = 1;
  SoftStop -> InactiveSS : [after(3, sec)]
  (default) -> InactiveSS
  InactiveSS -> SoftStop : [hasChangedFrom(WPActv, true)]
  data: WPActv input; SSActv output

== matlab function VSIGenLib/MinFunc ==
  data: Dist input; Min output; minIdx output
function [Min, minIdx] = fcn(Dist)
[Min, minIdx] = min(Dist);
